simulink model "Fig122"  (R2014a)
settings: Solver=ode3  StartTime=0.0  StopTime=.05  FixedStep=2e-6  RelTol=1e-3
undefined symbols (not defined in the file): fdesignblkfcn, gcbh
libraries: commchan3 x1
settings Model: Creator=Dennis Silage  LastModifiedBy=Silage
settings SolverCC: AutoInsertRateTranBlk=on
settings DataIOCC: SignalLoggingSaveFormat=ModelDataLogs
settings OptimizationCC: ExpressionDepthLimit=2147483647  InitFltsAndDblsToZero=on
settings DebuggingCC: UnderspecifiedInitializationDetection=Classic  FcnCallInpInsideContextMsg=UseLocalSettings  StateNameClashWarn=warning
settings GRTTargetCC: CombineOutputUpdateFcns=off  GRTInterface=on

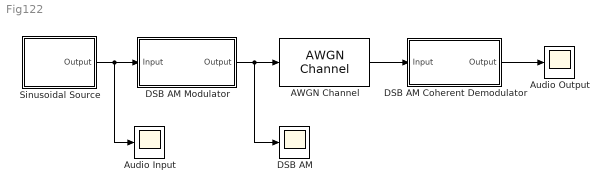
== system Fig122 ==
  AWGN Channel : commchan3/AWGN Channel  InputProcessing=Inherited (this choice will be removed - see release notes)  seed=randseed  noiseMode=Variance from mask  EbNodB=10  EsNodB=10  SNRdB=10  bitsPerSym=1  Ps=1  Tsym=1  variance=0
  Audio Output : Scope
      settings: MaxDataPoints=50000
  Audio Input : Scope
      settings: TimeRange=0.02  YMin=-2  YMax=2  SaveName=ScopeData2  MaxDataPoints=50000
  DSB AM : Scope
      settings: MaxDataPoints=50000
  DSB AM Coherent Demodulator : Subsystem
  DSB AM Modulator : Subsystem
  Sinusoidal Source : Subsystem
  wires:
  DSB AM Coherent Demodulator/1(Output) -> Audio Output/1
  AWGN Channel/1 -> DSB AM Coherent Demodulator/1(Input)
  DSB AM Modulator/1(Output) -> AWGN Channel/1, DSB AM/1
  Sinusoidal Source/1(Output) -> DSB AM Modulator/1(Input), Audio Input/1

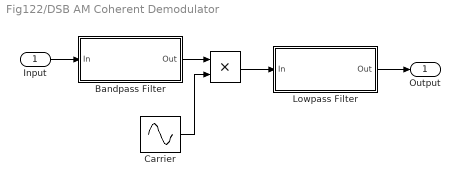
== system Fig122/DSB AM Coherent Demodulator ==
  Input : Inport
  " " : Product  RndMeth=Zero
  Bandpass Filter : Subsystem  DialogController=fdesignblkfcn  InitFcn=fdesignblkfcn(gcbh, {'InitFcn'});  mask(Bandpass Filter){}
      mask help: Design a bandpass filter
      settings: CopyFcn=fdesignblkfcn(gcbh, {'CopyFcn'});
      mask Help: helpview(mapfilelocation('dsp'), 'dspbandpassfilter');
      mask Display: disp('Bandpass');
  Carrier : Sin  Frequency=40000*pi  SampleTime=2e-6
  Lowpass Filter : Subsystem  DialogController=fdesignblkfcn  InitFcn=fdesignblkfcn(gcbh, {'InitFcn'});  mask(Lowpass Filter){}
      mask help: Design a lowpass filter
      settings: CopyFcn=fdesignblkfcn(gcbh, {'CopyFcn'});
      mask Help: helpview(mapfilelocation('dsp'), 'dsplowpassfilter');
      mask Display: disp('Lowpass')
  Output : Outport
  wires:
  Carrier/1 -> " "/2
  Input/1 -> Bandpass Filter/1(In)
  Bandpass Filter/1(Out) -> " "/1
  " "/1 -> Lowpass Filter/1(In)
  Lowpass Filter/1(Out) -> Output/1

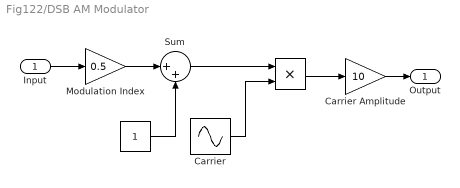
== system Fig122/DSB AM Modulator ==
  Input : Inport
  " " : Product  RndMeth=Zero
  "  " : Constant
  Carrier : Sin  Frequency=40000*pi  SampleTime=2e-6
  Carrier Amplitude : Gain  Gain=10
  Modulation Index : Gain  Gain=0.5
  Sum : Sum  Inputs=|++
  Output : Outport
  wires:
  Modulation Index/1 -> Sum/1
  "  "/1 -> Sum/2
  Sum/1 -> " "/1
  Carrier/1 -> " "/2
  " "/1 -> Carrier Amplitude/1
  Carrier Amplitude/1 -> Output/1
  Input/1 -> Modulation Index/1

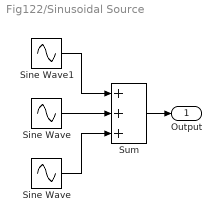
== system Fig122/Sinusoidal Source ==
  " Sine Wave " : Sin  Amplitude=0.2  Frequency=5000*pi  SampleTime=2e-6
  "Sine Wave " : Sin  Amplitude=0.5  Frequency=3000*pi  SampleTime=2e-6
  Sine Wave1 : Sin  Frequency=1000*pi  SampleTime=2e-6
  Sum : Sum  Inputs=+++
  Output : Outport
  wires:
  "Sine Wave "/1 -> Sum/2
  " Sine Wave "/1 -> Sum/3
  Sine Wave1/1 -> Sum/1
  Sum/1 -> Output/1

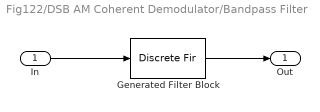
== system Fig122/DSB AM Coherent Demodulator/Bandpass Filter ==
  In : Inport
  Generated Filter Block : DiscreteFir  Tag=BlockMethodSubSystem  Coefficients=[9.9730629802221817e-05 -0.00092342257240285246 -0.00024971712843249217 -0.00017776552061724753 -0.00015764989760538211 -0.00013228098314588775 -9.7585515078851283e-05 -5.5794755472452894e-05 -1.0755393100970816e-05 3.3346362879018571e-05 7.2157178274305902e-05 0.0001020059357764694 0.0001199493175757586 0.00012469451246417186 0.00011630561243042238 9.6815822907801567e-05 6.9650774577275135e-05 3.9779443961024071e-05 1.2764941345747949e-05 -5.3245760916629994e-06 -9.2789715403540684e-06 5.0874146056731177e-06 3.9741927774859364e-05 9.4425830768060876e-05 0.00016568780718832256 0.00024745415641675415 0.00033072156945203768 0.00040478984648815715 0.00045741796981537894 0.00047675505000515544 0.00045198930254280523 0.00037537083146338087 0.00024269759462446376 5.5254250953072582e-05 -0.00018053922665988678 -0.00045191221953225192 -0.00074117541442917691 -0.0010255874203666364 -0.0012800758180382284 -0.0014776649874270159 -0.0015932355620549765 -0.0016051189399270457 -0.0014957451030598566 -0.0012605116481042972 -0.00089624048188281791 -0.00041871571709603962 0.0001488083922071879 0.00077451710486799359 0.0014177518687463796 0.0020311291895985339 0.0025655961390165741 0.0029734438975646837 0.0032126132110412847 0.0032500217528566521 0.0030653167759958342 0.0026533140096534446 0.0020257238140357903 0.0012112789285704758 0.00025486133108037329 -0.00078503906691319424 -0.0018399140029626878 -0.0028359085267028288 -0.0036992759689892006 -0.0043619874019106587 -0.0047672236586669614 -0.0048742369998279926 -0.0046623734986663591 -0.0041333755565430442 -0.0033122682038874748 -0.0022461618702814901 -0.001001745829690091 0.00033944303873015871 0.0016866367826637032 0.0029466907464906484 0.0040307989046071187 0.0048619030688714128 0.0053802885546074342 0.0055489179883982899 0.0053561415032876165 0.0048173320209192608 0.0039732245585755929 0.0028876532073956506 0.0016418158687906555 0.00032784640121340594 -0.00095750098564747631 -0.0021234880551177977 -0.0030888958823277551 -0.0037923530647280121 -0.0041953434885403191 -0.0042849316492205441 -0.0040750691913944842 -0.0036055041532678184 -0.0029366322394302779 -0.0021439601040045518 -0.0013106991680256128 -0.00051994452891565221 0.00015373738646277664 0.00065162412034628834 0.00093686202051887154 0.00099815549066095081 0.00085128526247643058 0.00053769967512305381 0.00012055665265052376 -0.00032161486538129127 -0.00070314239878761136 -0.00094049310137616 -0.00096179110688216266 -0.00071571815558929509 -0.00017897854315616717 0.00063886438867896602 0.0016933623198062248 0.0029066732017813306 0.0041720967483393637 0.0053622515051487936 0.006339675315516536 0.0069694025419798061 0.0071318552359890628 0.0067362677826073875 0.0057315970940456243 0.0041154158372120149 0.0019386782506428876 -0.0006932138312069657 -0.0036250963962085538 -0.0066599385621006618 -0.0095723530504789531 -0.012124923202340116 -0.014085856045680266 -0.015249890420709405 -0.015455047328653899 -0.014600216978018249 -0.012657147817021618 -0.0096776637055919421 -0.0057951688719930861 -0.0012203908979552191 0.0037705975210045161 0.0088530809280020911 0.013675296368757289 0.017883095792249382 0.021146494048320412 0.023185340352318284 0.023792543363090231 0.022852612287166021 0.020354421045382945 0.016396533454693173 0.011184602963287207 0.0050207544607591562 -0.0017145658829530591 -0.0085871124206285659 -0.01513806975699967 -0.02091599956104187 -0.025509295137516007 -0.028576341898875476 -0.029871548701952175 -0.029264919629007985 -0.026754054558265516 -0.022466788148920537 -0.016654652061162241 -0.0096772363303186115 -0.0019792378928172863 0.005939973601266889 0.01356020842733641 0.020376460310172366 0.025933940694734488 0.029860557957343506 0.031892154419095139 0.031892154419095139 0.029860557957343506 0.025933940694734488 0.020376460310172366 0.01356020842733641 0.005939973601266889 -0.0019792378928172863 -0.0096772363303186115 -0.016654652061162241 -0.022466788148920537 -0.026754054558265516 -0.029264919629007985 ...(+3469 chars)]  InputProcessing=Columns as channels (frame based)
  Out : Outport
  wires:
  In/1 -> Generated Filter Block/1
  Generated Filter Block/1 -> Out/1

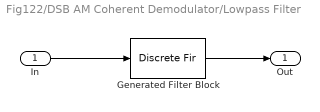
== system Fig122/DSB AM Coherent Demodulator/Lowpass Filter ==
  In : Inport
  Generated Filter Block : DiscreteFir  Tag=BlockMethodSubSystem  Coefficients=[0.00044688424903677106 -0.0002269396530557809 -0.00018451943627153849 -0.00015595035795888841 -0.00013646791283184617 -0.0001246465241434068 -0.00011742455149828799 -0.00011461457136234944 -0.00011404581504533614 -0.00011618396319684678 -0.00011931991748753365 -0.00012426924084328909 -0.00012955735971335457 -0.00013619047024976806 -0.00014280635094127646 -0.00015052585146214383 -0.00015802219409988673 -0.0001665199496377808 -0.00017459282401977651 -0.00018389146458461773 -0.00019197142054303413 -0.00020234599080188497 -0.00021081406592360434 -0.00022054990153549378 -0.00023055656785307081 -0.00024074142690237396 -0.00025022164847945358 -0.00026057564080612543 -0.00027084092162515776 -0.00028176463363290536 -0.00029204265390445831 -0.0003027929276505476 -0.0003130960486564258 -0.00032415884339311181 -0.00033483618018257381 -0.0003461278843951468 -0.0003567923926441329 -0.0003679559153175456 -0.00037843931310655522 -0.00038961077144177096 -0.00040001651108549863 -0.00041133352284568472 -0.00042174106434056581 -0.00043274120590049262 -0.00044320196345026434 -0.00045378754550774296 -0.00046373047688789694 -0.00047416645907563632 -0.00048386478734290363 -0.00049383371586610202 -0.00050314388141965336 -0.00051288097219187069 -0.00052184614563465111 -0.00053101571270462266 -0.00053932183118885922 -0.00054790215544784845 -0.00055564305632760142 -0.00056359759694367731 -0.00057057540248507807 -0.00057778139432284399 -0.00058399291698178757 -0.00059053918289884901 -0.00059606095604253825 -0.00060173343380842963 -0.00060647754956988679 -0.00061115449529462241 -0.00061490354832731387 -0.00061873668818275063 -0.00062148836217794097 -0.00062422588395112037 -0.00062593605203717525 -0.00062759123910731949 -0.00062809847420234222 -0.00062857390147677962 -0.00062799178405385488 -0.00062737338805300452 -0.00062559113654370646 -0.00062373231712993852 -0.00062071365232192191 -0.00061765134010304391 -0.00061335930115301968 -0.00060900295628483483 -0.00060344047198045234 -0.00059779203178158126 -0.00059103567158417017 -0.00058406439993106897 -0.00057594370329521133 -0.00056767228552877616 -0.00055819459984298673 -0.00054861017893497062 -0.00053789764356621645 -0.00052702895322409593 -0.00051498635375055125 -0.00050285889831332403 -0.00048960066149917811 -0.00047623307987323894 -0.00046172559324854167 -0.00044716053462067173 -0.00043146579533471271 -0.00041571994722393541 -0.00039886795051010987 -0.00038204742129230936 -0.00036419303329514227 -0.00034633221751640238 -0.00032748563815311778 -0.00030862001871527554 -0.00028883419808219764 -0.00026912563850305278 -0.00024847196170704565 -0.00022794842209710109 -0.0002065703305649941 -0.00018534583518564542 -0.0001633123600277989 -0.00014151444370250402 -0.00011893702330244087 -9.6634070736211766e-05 -7.364673169508128e-05 -5.1023986902019825e-05 -2.7731480269947641e-05 -4.8327210294805576e-06 1.8663627135460784e-05 4.1684730629644841e-05 6.5223736290382609e-05 8.8248248625158411e-05 0.00011167042948118653 0.00013452662795930559 0.00015772957989106074 0.00018028259784556519 0.00020314084296571154 0.00022524474813800509 0.00024756685056259806 0.00026911722815836403 0.00029081880585359515 0.00031164031157908178 0.00033254690536092113 0.00035250855079202827 0.00037247705372174501 0.00039144311985142143 0.00041037124323416716 0.00042821021654004289 0.00044591923459956126 0.00046249094898521747 0.0004788653655973133 0.00049404099972850252 0.00050891641504733167 0.00052256100576491085 0.00053587508624041618 0.00054788235304825434 0.00055951955578166729 0.00056978091253278001 0.0005796111929825226 0.0005880372387940553 0.00059597026374095272 0.00060244895841486744 0.00060842552600036317 0.00061290586482585607 0.00061681728085319657 0.00061920000782819803 0.00062100394237499853 0.00062125457480906581 0.00062090091552088531 0.00061898811319237312 0.00061642951979681262 0.00061229975659506802 0.00060750924113994395 0.00060116362790956206 0.00059414994147597919 0.0005855492289293311 0.000576310325967266 ...(+18783 chars)]  InputProcessing=Columns as channels (frame based)
  Out : Outport
  wires:
  In/1 -> Generated Filter Block/1
  Generated Filter Block/1 -> Out/1
